simulink model "slave"  (R2020a)
settings: Solver=FixedStepDiscrete  StartTime=0.0  StopTime=10.0  FixedStep=1000  RelTol=1e-3  EnableMultiTasking=on
settings Model: SILPILModeSetting=veronly  ExtModeTrigDuration=2  Creator=Yalda  LastModifiedBy=Yalda
settings OptimizationCC: DefaultParameterBehavior=Inlined  UseDivisionForNetSlopeComputation=on  GainParamInheritBuiltInType=on  UseFloatMulNetSlope=on  InlineInvariantSignals=on  PassReuseOutputArgsAs=Individual arguments  ZeroExternalMemoryAtStartup=off  ZeroInternalMemoryAtStartup=off  NoFixptDivByZeroProtection=on  EfficientFloat2IntCast=on  LifeSpan=1  MaxStackSize=64  OptimizeBlockOrder=speed  DifferentSizesBufferReuse=on  EfficientTunableParamExpr=on
settings DebuggingCC: ParameterTunabilityLossMsg=error
settings HardwareCC: ProdBitPerInt=16  ProdBitPerPointer=16  ProdBitPerSizeT=16  ProdBitPerPtrDiffT=16  ProdLargestAtomicFloat=None  ProdWordSize=8  ProdLongLongMode=on  ProdHWDeviceType=Atmel->AVR
settings SFSimCC: MATLABDynamicMemAlloc=off
settings RTWCC: SystemTargetFile=ert.tlc  HardwareBoard=Arduino Uno  TLCOptions=-aInlineSetEventsForThisBaseRateFcn=TLC_FALSE -aSuppressMultiTaskScheduler=TLC_FALSE -aRateBasedStepFcn=1  TemplateMakefile=ert_default_tmf  Toolchain=Arduino AVR  BuildConfiguration=Faster Runs
settings CodeAppCC: ForceParamTrailComments=on  IgnoreCustomStorageClasses=off  OperatorAnnotations=on  SimulinkDataObjDesc=on  SFDataObjDesc=on  CustomSymbolStrGlobalVar=rt$N$M  CustomSymbolStrType=$N$M  CustomSymbolStrFcn=$N$M$F  CustomSymbolStrMacro=$N$M  InsertBlockDesc=on
settings ERTTargetCC: IncludeMdlTerminateFcn=off  CombineSignalStateStructs=on  SupportAbsoluteTime=off  PurelyIntegerCode=on  SupportNonFinite=off  SupportComplex=off  SupportNonInlinedSFcns=on  ExtModeStaticAllocSize=250  InlinedParameterPlacement=NonHierarchical  ERTFilePackagingFormat=CompactWithDataFile

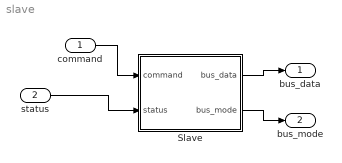
== system slave ==
  command : Inport
  status : Inport  Port=2
  Slave : Subsystem
  bus_data : Outport
  bus_mode : Outport  Port=2
  wires:
  command/1 -> Slave/1(command)
  status/1 -> Slave/2(status)
  Slave/1(bus_data) -> bus_data/1
  Slave/2(bus_mode) -> bus_mode/1

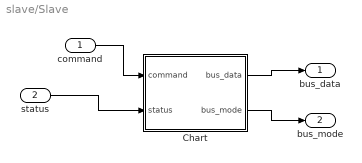
== system slave/Slave ==
  command : Inport
  status : Inport  Port=2
  Chart : Stateflow chart  TreatAsAtomicUnit=on
  bus_data : Outport
  bus_mode : Outport  Port=2
  wires:
  Chart/1(bus_data) -> bus_data/1
  status/1 -> Chart/2(status)
  command/1 -> Chart/1(command)
  Chart/2(bus_mode) -> bus_mode/1

== stateflow chart slave/Slave/Chart ==
  state free
  state checkAddr
  state getCommand
  state sending
  checkAddr -> free [order 1] : [command!=ID]
  (default) -> free : {bus_mode=0;}
  free -> checkAddr : [command==1]
  getCommand -> free [order 2] : [command==0]
  checkAddr -> sending [order 2] : [command==ID]{bus_mode=1; bus_data=status}
  sending -> getCommand : {bus_mode=0}
  getCommand -> sending [order 1] : [command!=0]{bus_mode=1;bus_data=status}
  data: command input uint8; status input uint8; bus_data output uint8; bus_mode output uint8; ID local uint8
